simulink model "differentiator"  (R2021a)
settings: Solver=FixedStepAuto  StartTime=0.0  StopTime=inf  FixedStep=0.1  RelTol=1e-3
libraries: robotlib x4, dspstat3 x1
settings Model: Creator=refulgent  LastModifiedBy=refulgent
settings OptimizationCC: EnhancedBackFolding=on  PassReuseOutputArgsAs=Individual arguments  ZeroExternalMemoryAtStartup=off  ZeroInternalMemoryAtStartup=off  MaxStackSize=64  OptimizeBlockOrder=speed  DifferentSizesBufferReuse=on  OptimizationCustomize=off  EfficientTunableParamExpr=on
settings DebuggingCC: ParameterTunabilityLossMsg=error
settings HardwareCC: ProdBitPerPointer=32  ProdBitPerSizeT=32  ProdBitPerPtrDiffT=32  ProdLargestAtomicFloat=None  ProdIntDivRoundTo=Undefined  ProdEndianess=Unspecified  ProdWordSize=32  ProdHWDeviceType=Generic->Unspecified (assume 32-bit Generic)
settings SFSimCC: MATLABDynamicMemAlloc=off
settings RTWCC: SystemTargetFile=ert.tlc  HardwareBoard=Robot Operating System (ROS)  TLCOptions="-aInlineSetEventsForThisBaseRateFcn=TLC_FALSE -aSuppressMultiTaskScheduler=TLC_FALSE  -aRateBasedStepFcn=0"  TemplateMakefile=ert_default_tmf  GenerateReport=on  Toolchain=Catkin  LaunchReport=on  TargetLang=C++  GenerateWebview=on
settings CodeAppCC: ForceParamTrailComments=on  IgnoreCustomStorageClasses=off  OperatorAnnotations=on  SimulinkDataObjDesc=on  SFDataObjDesc=on  InsertBlockDesc=on
settings ERTTargetCC: SupportContinuousTime=on

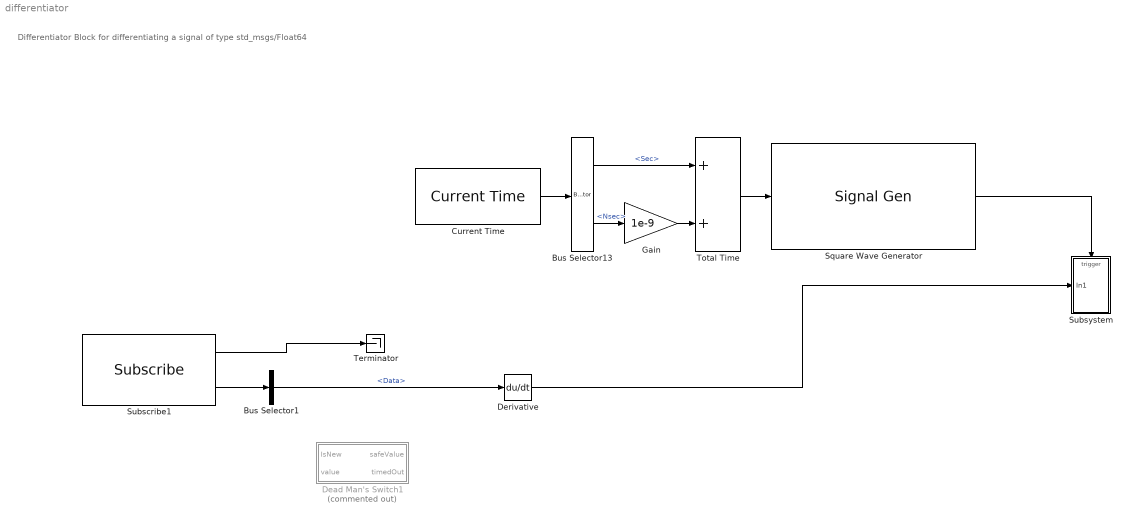
== system differentiator ==
  note: Differentiator Block for differentiating a signal of type std_msgs/Float64
  Bus Selector1 : BusSelector  OutputSignals=Data
  Bus Selector13 : BusSelector  OutputSignals=Sec,Nsec
  Current Time : robotlib/Current Time  OutputFormat=bus  SampleTime=-1  ModelName=differentiator
      settings: SourceProductBaseCode=RR
  Dead Man's Switch1 : Subsystem  Commented=on  TreatAsAtomicUnit=on  mask{stepSize=0.025, timeout=0.1}
      mask prompts: stepSize "Simulation step size"; timeout "Timeout (in seconds)"
      mask help: Interprets whether a new message has been recently received, and if so permits the data in 'value' to be passed through. Otherwise, 0 is outputted from 'safeValue'
      mask Help: Interprets whether a new message has been recently received, and if so permits the data in 'value' to be passed through. Otherwise, 0 is outputted from 'safeValue'
  Derivative : Derivative
  Gain : Gain  Gain=1e-9
  Square Wave Generator : SignalGenerator  WaveForm=square  TimeSource=Use external signal  Frequency=10
  Subscribe1 : robotlib/Subscribe  topicSource=Specify your own  topic=input  messageType=std_msgs/Float64  SampleTime=-1  legacyBusStruct=off  messageQueueLength=1
  Subsystem : Subsystem
  Terminator : Terminator
  Total Time : Sum
  wires:
  Subscribe1/2 -> Bus Selector1/1
  Subscribe1/1 -> Terminator/1
  Derivative/1 -> Subsystem/1(In1)
  Gain/1 -> Total Time/2
  Bus Selector13/2 -> Gain/1  "<Nsec>"
  Current Time/1 -> Bus Selector13/1
  Total Time/1 -> Square Wave Generator/1
  Square Wave Generator/1 -> Subsystem/Trigger
  Bus Selector13/1 -> Total Time/1  "<Sec>"
  Bus Selector1/1 -> Derivative/1  "<Data>"

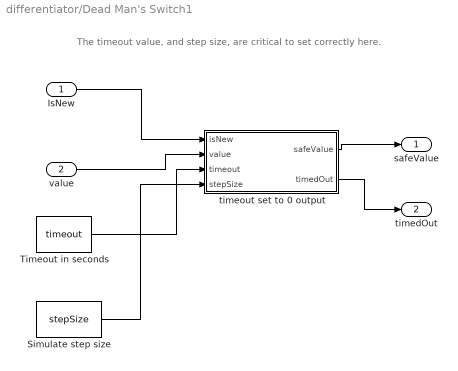
== system differentiator/Dead Man's Switch1 ==
  note: The timeout value, and step size, are critical to set correctly here.
  IsNew : Inport
  value : Inport  Port=2
  Simulate step size : Constant  Value=stepSize
  Timeout in seconds : Constant  Value=timeout
  timeout set to 0 output : MATLAB Function  TreatAsAtomicUnit=on
  safeValue : Outport  InitialOutput=[0]
  timedOut : Outport  Port=2  InitialOutput=[0]
  wires:
  Simulate step size/1 -> timeout set to 0 output/4(stepSize)
  timeout set to 0 output/2(timedOut) -> timedOut/1
  Timeout in seconds/1 -> timeout set to 0 output/3(timeout)
  value/1 -> timeout set to 0 output/2(value)
  timeout set to 0 output/1(safeValue) -> safeValue/1
  IsNew/1 -> timeout set to 0 output/1(isNew)

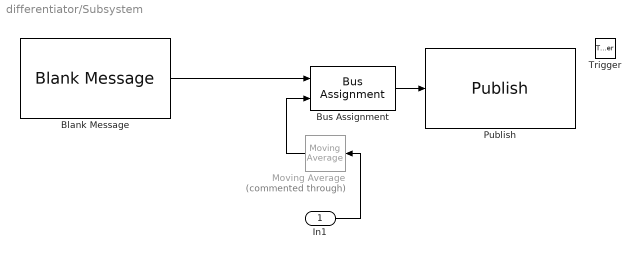
== system differentiator/Subsystem ==
  In1 : Inport
  Trigger : TriggerPort  VariantControl=(inherit)  PortDimensions=1
  Blank Message : robotlib/Blank Message  messageClass=Message  entityType=std_msgs/Float64  messageType=std_msgs/Float64  SampleTime=inf  legacyBusStruct=off
  Bus Assignment : BusAssignment  AssignedSignals=Data
  Moving Average : dspstat3/Moving Average  Commented=through  Method=Sliding window  ForgettingFactorPort=off  SpecifyWindowLength=on  WindowLength=20  ForgettingFactor=0.9  SimulateUsing=Code generation
  Publish : robotlib/Publish  topicSource=Specify your own  topic=derivative  messageType=std_msgs/Float64  legacyBusStruct=off  messageQueueLength=1
  wires:
  In1/1 -> Moving Average/1
  Moving Average/1 -> Bus Assignment/2
  Blank Message/1 -> Bus Assignment/1
  Bus Assignment/1 -> Publish/1

== matlab function differentiator/Dead Man's Switch1/timeout set to 0 output ==
  data: isNew input; safeValue output; value input; timeout input; timedOut output; stepSize input
function [safeValue,timedOut] = fcn(isNew,value,timeout,stepSize)
%#codegen
persistent sinceLastMsg
timedOut=true;
if isempty(sinceLastMsg)
    sinceLastMsg=(timeout/stepSize)+1;
end

safeValue=0;
% if no new message
% after timeout, we output 0
if( isNew == true )
    sinceLastMsg = 0;
else
    sinceLastMsg = sinceLastMsg+1;
end

% Note: we require step size as an input here, and depend on our
% system being executed at a regular rate, or bad things will happen
if( sinceLastMsg < timeout/stepSize )
    timedOut = false;
end
    
if( timedOut == false )
    safeValue = value;
end
